simulink model "autopilot13dng"  (Simulink 5.0)
settings: Solver=ode3  SolverMode=SingleTasking  StartTime=0.0  StopTime=150  FixedStep=.1  RelTol=1e-3
PreLoadFcn:
  | load autopilot_data.mat;
values from neighbouring files (symbols this model uses):
  a = 2.5348    [autopilot_data.mat]    (also in f14dat.m; f14def.m)
  alt_ic = 1200    [autopilot_data.mat]
  b = 64.13    [autopilot_data.mat]    (also in f14dat.m; f14def.m)
  Md = -6.8847    [autopilot_data.mat]    (also in f14dat.m; f14def.m)
  Mq = -0.0164275    [autopilot_data.mat]    (also in f14dat.m = -0.6571; f14def.m = -0.6571)
  Mw = -0.000148    [autopilot_data.mat]    (also in f14dat.m = -0.00592; f14def.m = -0.00592)
  Swg = 3    [autopilot_data.mat]    (also in f14dat.m; f14def.m)
  Ta = 0.05    [autopilot_data.mat]    (also in f14dat.m; f14def.m)
  Ts = 0.2    [autopilot_data.mat]    (also in f14dat.m = 0.1; f14def.m = 0.1)
  Uo = 689.4    [autopilot_data.mat]    (also in f14dat.m; f14def.m)
  Vto = 690.4    [autopilot_data.mat]    (also in f14dat.m; f14def.m)
  Zd = -63.9979    [autopilot_data.mat]    (also in f14dat.m; f14def.m)
  Zw = -0.0159625    [autopilot_data.mat]    (also in f14dat.m = -0.6385; f14def.m = -0.6385)
libraries: dnglibv1 x9, autopilot_plane x1, simulink x1
settings Model: Creator=pjackson  LastModifiedBy=kgondoly  RTWInlineParameters=on  RTWSystemTargetFile=ert.tlc  RTWTemplateMakefile=ert_default_tmf  RTWOptions="-aCombineOutputUpdateFcns=1 -aEnforceIntegerDowncast=1 -aExtMode=0 -aExtModeTesting=0 -aFoldNonRolledExpr=1 -aForceParamTrailComments=0 -aGenFloatMathFcnCalls=\"ANSI_C\" -aGenerateASAP2=0 -aGenerateComments=1 -aGenerateErtSFunction=0 -aGenerateReport=1 -aGenerateSampleERTMain=1 -aIgnoreCustomStorageClasses=0 -aIncDataTypeInIds=0 -aIncHierarchyInIds=0 -aIncludeMdlTerminateFcn=0 -aInitFltsAndDblsToZero=0 -aInlineInvariantSignals=1 -aInlinedPrmAccess=\"Literals\" -aInsertBlockDesc=0 -aLocalBlockOutputs=1 -aMatFileLogging=0 -aMaxRTWIdLen=31 -aMultiInstanceERTCode=0 -aPrefixModelToSubsysFcnNames=0 -aPurelyIntegerCode=0 -aRTWVerbose=1 -aRollThreshold=5 -aShowEliminatedStatements=0 -aSuppressErrorStatus=1 -aTargetOS=\"BareBoardExample\" -aZeroExternalMemoryAtStartup=0 -aZeroInternalMemoryAtStartup=0"

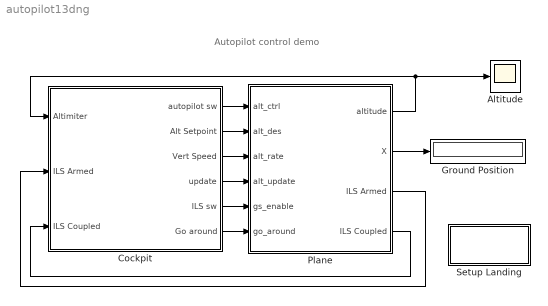
== system autopilot13dng ==
  note: Autopilot control demo
  Altitude : Scope
      settings: TickLabels=on  TimeRange=150  YMin=-100  YMax=1500
  Cockpit : Subsystem
  Ground Position : Display
  Plane : Subsystem  AncestorBlock=autopilot_plane/Plane
  Setup Landing : Subsystem
      settings: OpenFcn=alt_ic = 1200
      mask Display: disp('Setup\nLanding')
  wires:
  Cockpit/1(autopilot sw) -> Plane/1(alt_ctrl)
  Cockpit/2(Alt Setpoint) -> Plane/2(alt_des)
  Cockpit/3(Vert Speed) -> Plane/3(alt_rate)
  Cockpit/4(update) -> Plane/4(alt_update)
  Cockpit/5(ILS sw) -> Plane/5(gs_enable)
  Cockpit/6(Go around) -> Plane/6(go_around)
  Plane/1(altitude) -> Cockpit/1(Altimiter), Altitude/1
  Plane/3(ILS Armed) -> Cockpit/2(ILS Armed)
  Plane/4(ILS Coupled) -> Cockpit/3(ILS Coupled)
  Plane/2(X) -> Ground Position/1

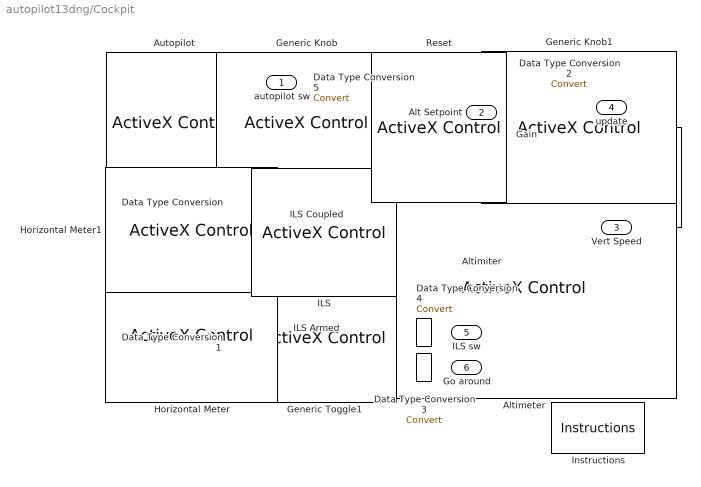
== system autopilot13dng/Cockpit ==
  Altimiter : Inport
  ILS Armed : Inport  Orientation=left  Port=2
  ILS Coupled : Inport  Orientation=left  Port=3
  Altimeter : dnglibv1/ActiveX Control  progid=air.airctrl.1  connect=input  input=altitude  init=hActx.displaymode=2;hActx.altthousandstyle=1;  inblock=on  border=on  dialOut=0  updateParam=0
  Autopilot : dnglibv1/ActiveX Control  progid=mwtoggle.togglectrl.1  connect=output  output=Value  dialOutEvent=Click  init=hActx.configuration='Toggle Switch\Bitmap Toggles\OnOff Switch';  inblock=on  border=on  dialOut=1  updateParam=0
  Data Type Conversion : DataTypeConversion  Orientation=left  SaturateOnIntegerOverflow=on
  Data Type Conversion1 : DataTypeConversion  Orientation=left  SaturateOnIntegerOverflow=on
  Data Type Conversion2 : DataTypeConversion  DataType=boolean  SaturateOnIntegerOverflow=on
  Data Type Conversion3 : DataTypeConversion  DataType=boolean  SaturateOnIntegerOverflow=on
  Data Type Conversion4 : DataTypeConversion  DataType=boolean  SaturateOnIntegerOverflow=on
  Data Type Conversion5 : DataTypeConversion  Orientation=up  DataType=boolean  SaturateOnIntegerOverflow=on
  Gain : Gain  Gain=-1  SaturateOnIntegerOverflow=on
  Generic Knob : dnglibv1/ActiveX Control  progid=mwknob.knobctrl.1  connect=output  output=KnobValue  dialOutEvent=Turn Click  init=hActx.MouseControl=2;  inblock=on  border=on  dialOut=12000  updateParam=0
  Generic Knob1 : dnglibv1/ActiveX Control  progid=mwknob.knobctrl.1  connect=output  output=KnobValue  dialOutEvent=Turn Click  init=hActx.MouseControl=2;  inblock=on  border=on  dialOut=750  updateParam=0
  Generic Toggle1 : dnglibv1/ActiveX Control  progid=mwtoggle.togglectrl.1  connect=output  output=Value  dialOutEvent=Click  inblock=on  border=on  dialOut=0  updateParam=0
  Horizontal Meter : dnglibv1/ActiveX Control  Orientation=down  progid=MWLED.ledctrl.1  connect=input  input=Value  init=hActx.configuration='LED\Sets\Horizontal\Rectangle Horizontal Bitmaps';hActx.Mode=0;hActx.value=0;hActx.Mode=0;hActx.MouseControl=0;  inblock=on  border=on  dialOut=0  updateParam=0
  Horizontal Meter1 : dnglibv1/ActiveX Control  Orientation=down  progid=MWLED.ledctrl.1  connect=input  input=Value  init=hActx.configuration='LED\Sets\Horizontal\Rectangle Horizontal Bitmaps';hActx.Mode=0;hActx.value=0;hActx.Mode=0;hActx.MouseControl=0;  inblock=on  border=on  dialOut=0  updateParam=0
  ILS : dnglibv1/ActiveX Control  progid=mwtoggle.togglectrl.1  connect=output  output=Value  dialOutEvent=Click  init=hActx.configuration='Toggle Switch\Bitmap Toggles\OnOff Switch';  inblock=on  border=on  dialOut=1  updateParam=0
  Instructions : autopilot_plane/Instructions
  Reset : dnglibv1/ActiveX Control  progid=mwtoggle.togglectrl.1  connect=output  output=Value  dialOutEvent=Click  inblock=on  border=on  dialOut=0  updateParam=0
  autopilot sw : Outport
  Alt Setpoint : Outport  Port=2
  Vert Speed : Outport  Port=3
  update : Outport  Port=4
  ILS sw : Outport  Port=5
  Go around : Outport  Port=6
  wires:
  ILS Coupled/1 -> Data Type Conversion/1
  ILS Armed/1 -> Data Type Conversion1/1
  Altimiter/1 -> Altimeter/1
  Generic Knob1/1 -> Vert Speed/1
  Generic Knob/1 -> Alt Setpoint/1
  Reset/1 -> Gain/1
  Autopilot/1 -> Data Type Conversion5/1
  ILS/1 -> Data Type Conversion4/1
  Generic Toggle1/1 -> Data Type Conversion3/1
  Gain/1 -> Data Type Conversion2/1
  Data Type Conversion/1 -> Horizontal Meter/1
  Data Type Conversion1/1 -> Horizontal Meter1/1
  Data Type Conversion2/1 -> update/1
  Data Type Conversion3/1 -> Go around/1
  Data Type Conversion4/1 -> ILS sw/1
  Data Type Conversion5/1 -> autopilot sw/1

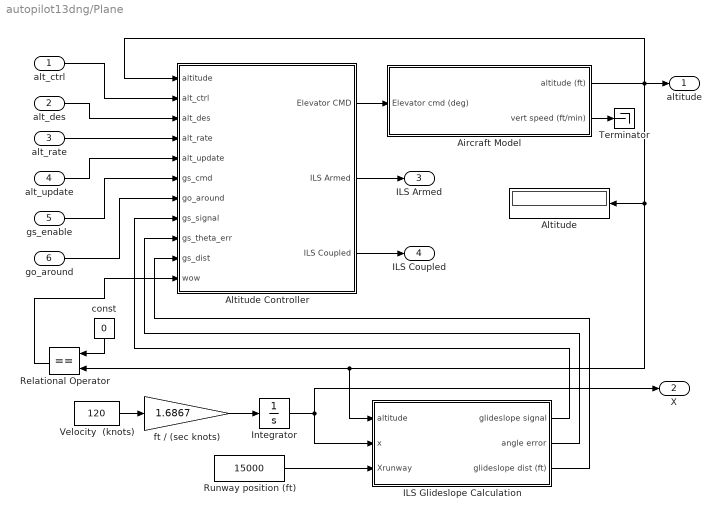
== system autopilot13dng/Plane ==
  alt_ctrl : Inport
  alt_des : Inport  Port=2
  alt_rate : Inport  Port=3
  alt_update : Inport  Port=4
  gs_enable : Inport  Port=5
  go_around : Inport  Port=6
  Aircraft Model : Subsystem
  Altitude : Display
  Altitude Controller : Subsystem
  ILS Glideslope Calculation : Subsystem
  Integrator : Integrator
  Relational Operator : RelationalOperator  Orientation=left  Operator===  InputSameDT=on
  Runway position (ft) : Constant  Value=15000
  Terminator : Terminator
  Velocity  (knots) : Constant  Value=120
  const : Constant  Orientation=down  Value=0
  ft / (sec knots) : Gain  Gain=1.6867  SaturateOnIntegerOverflow=on
  altitude : Outport
  X : Outport  Port=2
  ILS Armed : Outport  Port=3
  ILS Coupled : Outport  Port=4
  wires:
  const/1 -> Relational Operator/1
  Relational Operator/1 -> Altitude Controller/11(wow)
  Altitude Controller/3(ILS Coupled) -> ILS Coupled/1
  Altitude Controller/2(ILS Armed) -> ILS Armed/1
  go_around/1 -> Altitude Controller/7(go_around)
  gs_enable/1 -> Altitude Controller/6(gs_cmd)
  alt_update/1 -> Altitude Controller/5(alt_update)
  alt_rate/1 -> Altitude Controller/4(alt_rate)
  alt_des/1 -> Altitude Controller/3(alt_des)
  alt_ctrl/1 -> Altitude Controller/2(alt_ctrl)
  Aircraft Model/2(vert speed (ft/min)) -> Terminator/1
  ILS Glideslope Calculation/1(glideslope signal) -> Altitude Controller/8(gs_signal)
  ILS Glideslope Calculation/3(glideslope dist (ft)) -> Altitude Controller/10(gs_dist)
  ILS Glideslope Calculation/2(angle error) -> Altitude Controller/9(gs_theta_err)
  Runway position (ft)/1 -> ILS Glideslope Calculation/3(Xrunway)
  Integrator/1 -> X/1, ILS Glideslope Calculation/2(x)
  Velocity  (knots)/1 -> ft / (sec knots)/1
  ft / (sec knots)/1 -> Integrator/1
  Aircraft Model/1(altitude (ft)) -> Relational Operator/2, ILS Glideslope Calculation/1(altitude), Altitude/1, Altitude Controller/1(altitude), altitude/1
  Altitude Controller/1(Elevator CMD) -> Aircraft Model/1(Elevator cmd (deg))

== system autopilot13dng/Setup Landing ==

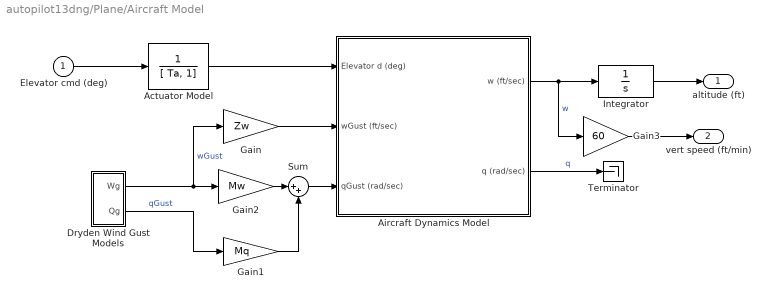
== system autopilot13dng/Plane/Aircraft Model ==
  Elevator cmd (deg) : Inport
  Actuator Model : TransferFcn  Denominator=[ Ta, 1]
  Aircraft Dynamics Model : Subsystem
  Dryden Wind Gust Models : Subsystem
  Gain : Gain  Gain=Zw  SaturateOnIntegerOverflow=on
  Gain1 : Gain  Gain=Mq  SaturateOnIntegerOverflow=on
  Gain2 : Gain  Gain=Mw  SaturateOnIntegerOverflow=on
  Gain3 : Gain  Gain=60  SaturateOnIntegerOverflow=on
  Integrator : Integrator  InitialCondition=alt_ic  LimitOutput=on  LowerSaturationLimit=0
  Sum : Sum  Inputs=|++  SaturateOnIntegerOverflow=on  InputSameDT=on
  Terminator : Terminator
  altitude (ft) : Outport
  vert speed (ft/min) : Outport  Port=2
  wires:
  Sum/1 -> Aircraft Dynamics Model/3(qGust (rad/sec))
  Gain/1 -> Aircraft Dynamics Model/2(wGust (ft/sec))
  Gain2/1 -> Sum/1
  Dryden Wind Gust Models/2(Qg) -> Gain1/1  "qGust"
  Dryden Wind Gust Models/1(Wg) -> Gain/1, Gain2/1  "wGust"
  Gain1/1 -> Sum/2
  Actuator Model/1 -> Aircraft Dynamics Model/1(Elevator d (deg))
  Aircraft Dynamics Model/1(w (ft/sec)) -> Integrator/1, Gain3/1  "w"
  Elevator cmd (deg)/1 -> Actuator Model/1
  Aircraft Dynamics Model/2(q (rad/sec)) -> Terminator/1  "q"
  Integrator/1 -> altitude (ft)/1
  Gain3/1 -> vert speed (ft/min)/1

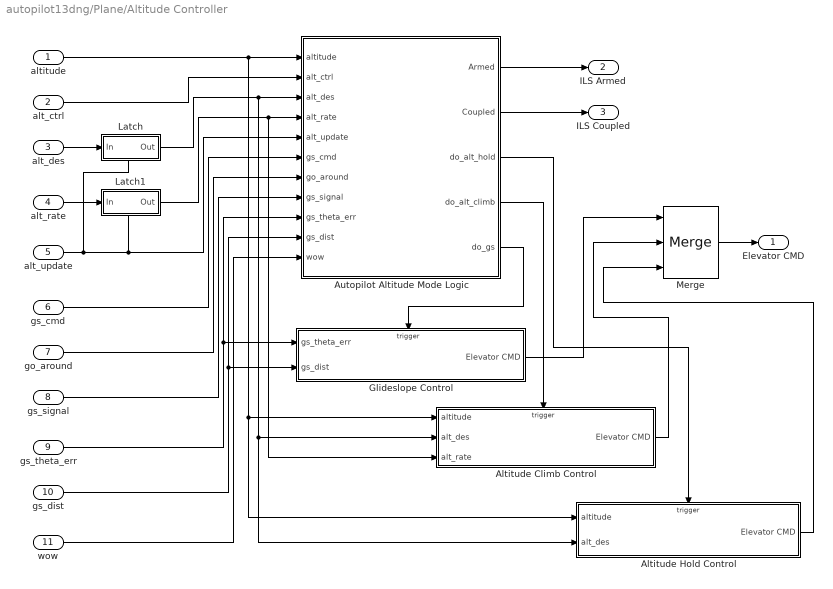
== system autopilot13dng/Plane/Altitude Controller ==
  altitude : Inport  SampleTime=Ts
  alt_ctrl : Inport  Port=2  SampleTime=Ts
  alt_des : Inport  Port=3  SampleTime=Ts
  alt_rate : Inport  Port=4  SampleTime=Ts
  alt_update : Inport  Port=5  SampleTime=Ts
  gs_cmd : Inport  Port=6  SampleTime=Ts
  go_around : Inport  Port=7  SampleTime=Ts
  gs_signal : Inport  Port=8  SampleTime=Ts
  gs_theta_err : Inport  Port=9  SampleTime=Ts
  gs_dist : Inport  Port=10  SampleTime=Ts
  wow : Inport  Port=11  SampleTime=Ts
  Altitude Climb Control : Subsystem  TreatAsAtomicUnit=on
  Altitude Hold Control : Subsystem  TreatAsAtomicUnit=on
  Autopilot Altitude Mode Logic : Stateflow chart
  Glideslope Control : Subsystem  TreatAsAtomicUnit=on
  Latch : Subsystem  TreatAsAtomicUnit=on
      settings: RTWSystemCode=Inline
  Latch1 : Subsystem  TreatAsAtomicUnit=on
      settings: RTWSystemCode=Inline
  Merge : Merge  Inputs=3
  Elevator CMD : Outport
  ILS Armed : Outport  Port=2
  ILS Coupled : Outport  Port=3
  wires:
  Autopilot Altitude Mode Logic/2(Coupled) -> ILS Coupled/1
  wow/1 -> Autopilot Altitude Mode Logic/11(wow)
  Latch1/1(Out) -> Autopilot Altitude Mode Logic/4(alt_rate), Altitude Climb Control/3(alt_rate)
  alt_rate/1 -> Latch1/1(In)
  Latch/1(Out) -> Autopilot Altitude Mode Logic/3(alt_des), Altitude Climb Control/2(alt_des), Altitude Hold Control/2(alt_des)
  alt_des/1 -> Latch/1(In)
  Autopilot Altitude Mode Logic/1(Armed) -> ILS Armed/1
  gs_dist/1 -> Autopilot Altitude Mode Logic/10(gs_dist), Glideslope Control/2(gs_dist)
  gs_theta_err/1 -> Autopilot Altitude Mode Logic/9(gs_theta_err), Glideslope Control/1(gs_theta_err)
  gs_signal/1 -> Autopilot Altitude Mode Logic/8(gs_signal)
  go_around/1 -> Autopilot Altitude Mode Logic/7(go_around)
  gs_cmd/1 -> Autopilot Altitude Mode Logic/6(gs_cmd)
  alt_update/1 -> Latch/Enable, Autopilot Altitude Mode Logic/5(alt_update), Latch1/Enable
  alt_ctrl/1 -> Autopilot Altitude Mode Logic/2(alt_ctrl)
  altitude/1 -> Autopilot Altitude Mode Logic/1(altitude), Altitude Climb Control/1(altitude), Altitude Hold Control/1(altitude)
  Merge/1 -> Elevator CMD/1
  Altitude Hold Control/1(Elevator CMD) -> Merge/3
  Altitude Climb Control/1(Elevator CMD) -> Merge/2
  Glideslope Control/1(Elevator CMD) -> Merge/1
  Autopilot Altitude Mode Logic/3(do_alt_hold) -> Altitude Hold Control/Trigger
  Autopilot Altitude Mode Logic/4(do_alt_climb) -> Altitude Climb Control/Trigger
  Autopilot Altitude Mode Logic/5(do_gs) -> Glideslope Control/Trigger

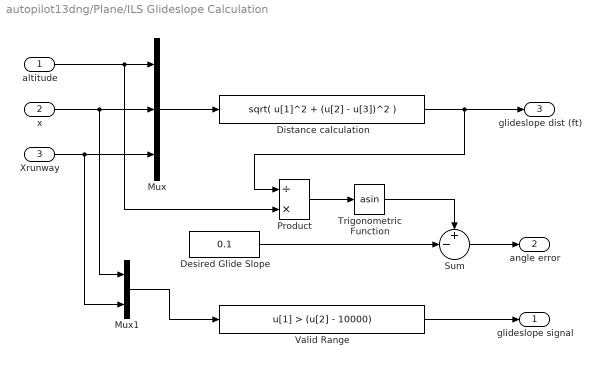
== system autopilot13dng/Plane/ILS Glideslope Calculation ==
  altitude : Inport
  x : Inport  Port=2
  Xrunway : Inport  Port=3
  Desired Glide Slope : Constant  Value=0.1
  Distance calculation : Fcn  Expr=sqrt( u[1]^2 + (u[2] - u[3])^2 )
  Mux : Mux  Inputs=3
  Mux1 : Mux  Inputs=2
  Product : Product  Inputs=/*  SaturateOnIntegerOverflow=on  InputSameDT=on
  Sum : Sum  Inputs=+-|  SaturateOnIntegerOverflow=on  InputSameDT=on
  Trigonometric Function : Trigonometry  Operator=asin
  Valid Range : Fcn  Expr=u[1] > (u[2] - 10000)
  glideslope signal : Outport
  angle error : Outport  Port=2
  glideslope dist (ft) : Outport  Port=3
  wires:
  Valid Range/1 -> glideslope signal/1
  Mux1/1 -> Valid Range/1
  Trigonometric Function/1 -> Sum/1
  Product/1 -> Trigonometric Function/1
  Sum/1 -> angle error/1
  Desired Glide Slope/1 -> Sum/2
  Xrunway/1 -> Mux1/2, Mux/3
  x/1 -> Mux1/1, Mux/2
  Distance calculation/1 -> Product/1, glideslope dist (ft)/1
  altitude/1 -> Product/2, Mux/1
  Mux/1 -> Distance calculation/1

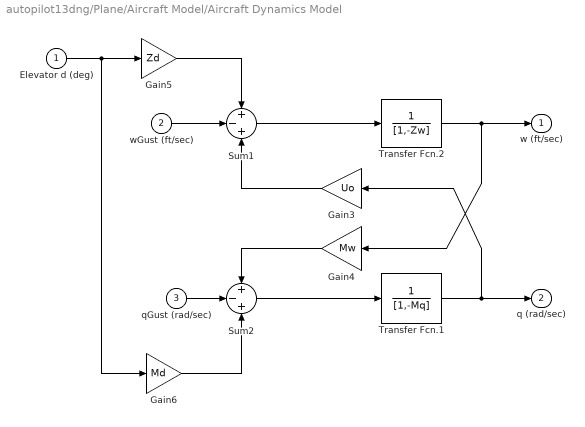
== system autopilot13dng/Plane/Aircraft Model/Aircraft Dynamics Model ==
  Elevator d (deg) : Inport
  wGust (ft/sec) : Inport  Port=2
  qGust (rad/sec) : Inport  Port=3
  Gain3 : Gain  Orientation=left  Gain=Uo  SaturateOnIntegerOverflow=on
  Gain4 : Gain  Orientation=left  Gain=Mw  SaturateOnIntegerOverflow=on
  Gain5 : Gain  Gain=Zd  SaturateOnIntegerOverflow=on
  Gain6 : Gain  Gain=Md  SaturateOnIntegerOverflow=on
  Sum1 : Sum  Inputs=+-+  SaturateOnIntegerOverflow=on  InputSameDT=on
  Sum2 : Sum  Inputs=+-+  SaturateOnIntegerOverflow=on  InputSameDT=on
  Transfer Fcn.1 : TransferFcn  Denominator=[1,-Mq]
  Transfer Fcn.2 : TransferFcn  Denominator=[1,-Zw]
  w (ft/sec) : Outport  InitialOutput=0
  q (rad/sec) : Outport  Port=2  InitialOutput=0
  wires:
  Elevator d (deg)/1 -> Gain6/1, Gain5/1
  wGust (ft/sec)/1 -> Sum1/2
  Gain4/1 -> Sum2/1
  Sum1/1 -> Transfer Fcn.2/1
  Sum2/1 -> Transfer Fcn.1/1
  qGust (rad/sec)/1 -> Sum2/2
  Gain3/1 -> Sum1/3
  Gain5/1 -> Sum1/1
  Gain6/1 -> Sum2/3
  Transfer Fcn.1/1 -> Gain3/1, q (rad/sec)/1
  Transfer Fcn.2/1 -> Gain4/1, w (ft/sec)/1

== system autopilot13dng/Plane/Aircraft Model/Dryden Wind Gust Models ==
  Band-Limited White Noise : simulink/Sources/Band-Limited White Noise  Cov=1  Ts=0.2  seed=[23341]
  Q-gust model : TransferFcn  Numerator=pi/(4*b)*[1 0]  Denominator=[1 pi*Vto/(4*b)]
  W-gust model : TransferFcn  Numerator=Swg/sqrt(a^3)*[sqrt(3)*a,1]  Denominator=[1 (2/a) 1/a^2]
  Wg : Outport  InitialOutput=0
  Qg : Outport  Port=2  InitialOutput=0
  wires:
  W-gust model/1 -> Q-gust model/1, Wg/1
  Q-gust model/1 -> Qg/1
  Band-Limited White Noise/1 -> W-gust model/1

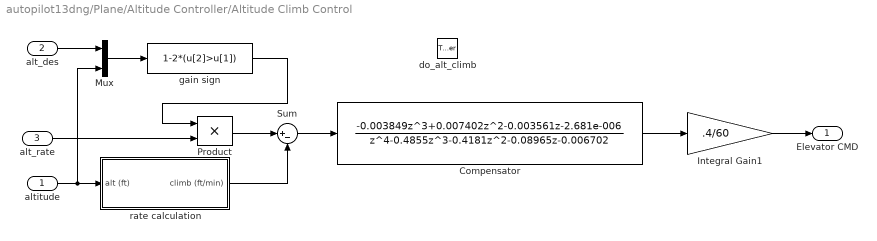
== system autopilot13dng/Plane/Altitude Controller/Altitude Climb Control ==
  altitude : Inport
  alt_des : Inport  Port=2
  alt_rate : Inport  Port=3
  do_alt_climb : TriggerPort  TriggerType=function-call
  Compensator : DiscreteTransferFcn  Numerator="[-0.003849   0.007402  -0.003561 -2.681e-006]"  Denominator="[1 -0.4855  -0.4181 -0.08965  -0.006702]"  SampleTime=-1
  Integral Gain1 : Gain  Gain=.4/60  SaturateOnIntegerOverflow=on
  Mux : Mux  Inputs=2
  Product : Product  SaturateOnIntegerOverflow=on  InputSameDT=on
  Sum : Sum  Inputs=|+-  SaturateOnIntegerOverflow=on  InputSameDT=on
  gain sign : Fcn  Expr=1-2*(u[2]>u[1])
  rate calculation : Subsystem
  Elevator CMD : Outport
  wires:
  Integral Gain1/1 -> Elevator CMD/1
  Compensator/1 -> Integral Gain1/1
  gain sign/1 -> Product/1
  alt_rate/1 -> Product/2
  Product/1 -> Sum/1
  Mux/1 -> gain sign/1
  alt_des/1 -> Mux/1
  altitude/1 -> Mux/2, rate calculation/1(alt (ft))
  rate calculation/1(climb (ft/min)) -> Sum/2
  Sum/1 -> Compensator/1

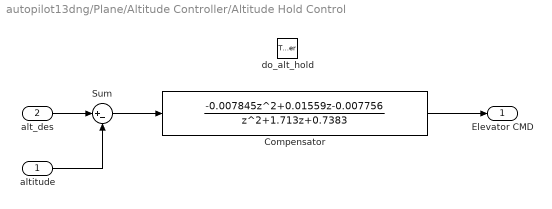
== system autopilot13dng/Plane/Altitude Controller/Altitude Hold Control ==
  altitude : Inport
  alt_des : Inport  Port=2
  do_alt_hold : TriggerPort  TriggerType=function-call
  Compensator : DiscreteTransferFcn  Numerator="[-0.007845  0.01559 -0.007756]"  Denominator="[1 1.713  0.7383]"  SampleTime=-1
  Sum : Sum  Inputs=|+-  SaturateOnIntegerOverflow=on  InputSameDT=on
  Elevator CMD : Outport
  wires:
  Sum/1 -> Compensator/1
  Compensator/1 -> Elevator CMD/1
  altitude/1 -> Sum/2
  alt_des/1 -> Sum/1

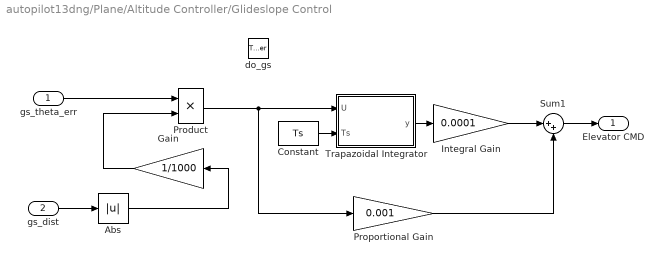
== system autopilot13dng/Plane/Altitude Controller/Glideslope Control ==
  gs_theta_err : Inport
  gs_dist : Inport  Port=2
  do_gs : TriggerPort  TriggerType=function-call
  Abs : Abs  SaturateOnIntegerOverflow=on
  Constant : Constant  Value=Ts
  Gain : Gain  Orientation=left  Gain=1/1000  SaturateOnIntegerOverflow=on
  Integral Gain : Gain  Gain=0.0001  SaturateOnIntegerOverflow=on
  Product : Product  SaturateOnIntegerOverflow=on  InputSameDT=on
  Proportional Gain : Gain  Gain=0.001  SaturateOnIntegerOverflow=on
  Sum1 : Sum  Inputs=|++  SaturateOnIntegerOverflow=on  InputSameDT=on
  Trapazoidal Integrator : Subsystem
      mask Type: No Time Trapazoid Integrator
      mask Description: Discrete-time integrator with no dependence on absolute time.  U is the input value and Ts is the discrete sample time.
      mask Display:
      | disp(sprintf('T(z+1)\n-----\n2(z-1)'))
      | port_label('input',1,'U');
      | port_label('input',2,'Ts');
  Elevator CMD : Outport
  wires:
  Constant/1 -> Trapazoidal Integrator/2(Ts)
  gs_dist/1 -> Abs/1
  Abs/1 -> Gain/1
  Gain/1 -> Product/2
  gs_theta_err/1 -> Product/1
  Product/1 -> Trapazoidal Integrator/1(U), Proportional Gain/1
  Trapazoidal Integrator/1(y) -> Integral Gain/1
  Proportional Gain/1 -> Sum1/2
  Integral Gain/1 -> Sum1/1
  Sum1/1 -> Elevator CMD/1

== system autopilot13dng/Plane/Altitude Controller/Latch ==
  In : Inport
  Enable : EnablePort
  Out : Outport  InitialOutput=alt_ic
  wires:
  In/1 -> Out/1

== system autopilot13dng/Plane/Altitude Controller/Latch1 ==
  In : Inport
  Enable : EnablePort
  Out : Outport  InitialOutput=10000
  wires:
  In/1 -> Out/1

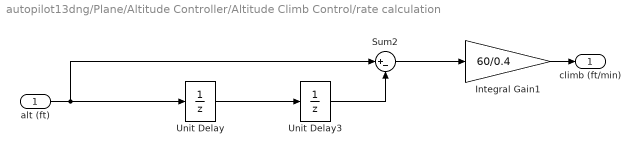
== system autopilot13dng/Plane/Altitude Controller/Altitude Climb Control/rate calculation ==
  alt (ft) : Inport
  Integral Gain1 : Gain  Gain=60/0.4  SaturateOnIntegerOverflow=on
  Sum2 : Sum  Inputs=|+-  SaturateOnIntegerOverflow=on  InputSameDT=on
  Unit Delay : UnitDelay  X0=10000  SampleTime=-1
  Unit Delay3 : UnitDelay  X0=10000  SampleTime=-1
  climb (ft/min) : Outport
  wires:
  Integral Gain1/1 -> climb (ft/min)/1
  Sum2/1 -> Integral Gain1/1
  Unit Delay3/1 -> Sum2/2
  alt (ft)/1 -> Sum2/1, Unit Delay/1
  Unit Delay/1 -> Unit Delay3/1

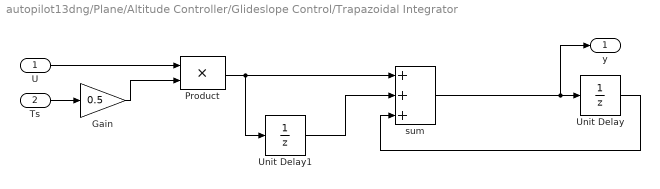
== system autopilot13dng/Plane/Altitude Controller/Glideslope Control/Trapazoidal Integrator ==
  U : Inport
  Ts : Inport  Port=2
  Gain : Gain  Gain=0.5
  Product : Product  InputSameDT=on
  Unit Delay : UnitDelay  SampleTime=-1
  Unit Delay1 : UnitDelay  SampleTime=-1
  sum : Sum  Inputs=+++  InputSameDT=on
  y : Outport
  wires:
  Product/1 -> sum/1, Unit Delay1/1
  Unit Delay1/1 -> sum/2
  sum/1 -> Unit Delay/1, y/1
  Unit Delay/1 -> sum/3
  U/1 -> Product/1
  Gain/1 -> Product/2
  Ts/1 -> Gain/1

== stateflow chart Plane/Altitude Controller/Autopilot Altitude Mode Logic ==
  settings: updateMethod=DISCRETE  sampleTime=Ts
  state out = alt_capture() [function]
    (default) -> (junction 19) : {out = abs(altitude - alt_des) < 30*Ts*(alt_rate / 60);}
  state GS [parallel]
    state Off
    state Active
      state Armed
      state Coupled /du: do_gs;
        state Around
        state Norm
        (default) -> Norm
        Norm -> Around : [go_around]
      Armed -> Coupled /du: do_gs; : [gs_coupled()]
      (default) -> Armed
    GS.Active -> Off : [~gs_cmd | ...
        |  ~gs_signal | wow]
    (default) -> Off
    Off -> GS.Active : [gs_cmd & ...
        | gs_signal & ~wow]
  state out = gs_coupled() [function]
    (default) -> (junction 18) : {out = gs_dist<10000 & gs_theta_err>0;}
  note: Glideslope
  state Altitude [parallel]
    state Disabled
    state Active
      state Climb_Rate
        du: do_alt_climb;
      state Hold
        du: do_alt_hold;
      Hold -> Climb_Rate : [abs(altitude-alt_des) >1500]
      Climb_Rate -> Hold : [alt_capture()]
    Disabled -> Hold : [alt_ctrl & ~wow & ...
        | ~in(GS.Active.Coupled)]
    (default) -> Disabled
    Altitude.Active -> Disabled : [in(GS.Active.Coupled) | ...
        | ~alt_ctrl | wow]
  data: out function_output; out function_output; altitude input double; alt_ctrl input boolean; alt_des input double; alt_rate input double; alt_update input boolean; gs_cmd input boolean; go_around input boolean; gs_signal input double; gs_theta_err input double; gs_dist input double; Ts constant double =0.2; Armed output State; Coupled output State; wow input boolean
  events: do_alt_hold output FUNCTION_CALL_EVENT; do_alt_climb output FUNCTION_CALL_EVENT; do_gs output FUNCTION_CALL_EVENT
